simulink model "buck_converter_with_Hysteresis_control"  (R2015a)
settings: Solver=ode45  StartTime=0.0  StopTime=3/1000  MaxStep=1/1000000  RelTol=1e-3
libraries: powerlib x9
settings Model: Creator=Windows 10  LastModifiedBy=Windows 10

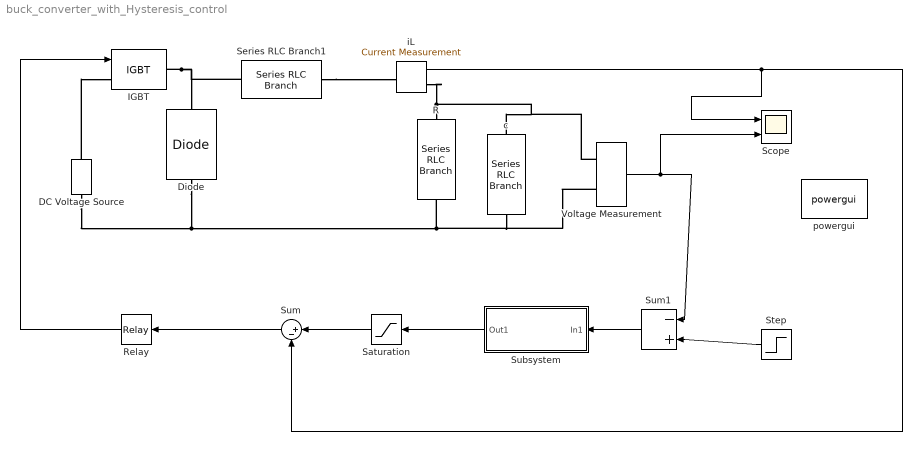
== system buck_converter_with_Hysteresis_control ==
  DC Voltage Source : powerlib/Electrical Sources/DC Voltage Source  Amplitude=100  Measurements=None
  Diode : powerlib/Power Electronics/Diode  Ron=0.001  Lon=0  Vf=0.8  IC=0  UseSnubber=off  Rs=500  Cs=250e-9  Measurements=off
  IGBT : powerlib/Power Electronics/IGBT  Ron=0.001  Lon=0  Vf=1  Tf=1e-6  Tt=2e-6  IC=0  Rs=1e5  Cs=inf  Measurements=off
  R : powerlib/Elements/Series RLC Branch  LConnTagsString=__new0  RConnTagsString=__new0  BranchType=R  Resistance=5  Inductance=1e-3  SetiL0=off  InitialCurrent=0  Capacitance=1e-6  Setx0=off  InitialVoltage=0  Measurements=None
  Relay : Relay  OnSwitchValue=0.5  OffSwitchValue=-0.5
  Saturation : Saturate  UpperLimit=20  LowerLimit=-20
  Scope : Scope  NumInputPorts=2
      settings: YMin=-5~-5  YMax=5~5
  Series RLC Branch1 : powerlib/Elements/Series RLC Branch  LConnTagsString=__new0  RConnTagsString=__new0  BranchType=L  Resistance=5  Inductance=0.01e-3  SetiL0=off  InitialCurrent=0  Capacitance=1e-6  Setx0=off  InitialVoltage=0  Measurements=Branch voltage
  Step : Step  Time=1.5/1000  Before=50  After=80  SampleTime=0
  Subsystem : Subsystem
  Sum : Sum  Inputs=|+-
  Sum1 : Sum  Inputs=|-+
  Voltage Measurement : powerlib/Measurements/Voltage Measurement  PhasorSimulation=off  OutputType=Complex  PSBequivalent=0
  c : powerlib/Elements/Series RLC Branch  LConnTagsString=__new0  RConnTagsString=__new0  BranchType=C  Resistance=5  Inductance=1e-3  SetiL0=off  InitialCurrent=0  Capacitance=20e-6  Setx0=off  InitialVoltage=0  Measurements=None
  iL : powerlib/Measurements/Current Measurement  PhasorSimulation=off  OutputType=Complex  PSBequivalent=0
  powergui : powerlib/powergui  Priority=1  SimulationMode=Continuous  SolverType=Tustin/Backward Euler (TBE)  SampleTime=50e-6  frequency=60  SPID=off  DisableSnubberDevices=off  DisableRonSwitches=off  DisableVfSwitches=off  SwTol=0  DisplayEquations=off  Interpol=off  methode=off  Ts=100  FunctionMessages=off  echomessages=off  HookPort=off  EnableUseOfTLC=off  x0status=blocks  frequencyindice=0  Pbase=100e6  ErrMax=1e-4  Iterations=50  UnitsV=kV  UnitsW=MW  buscounter=0  RestoreLinks=warning  ResistiveCurrentMeasurement=off  Frange=[0:2:500]  Ylog=off  Xlog=on  ShowGrid=off  save=off  variable=ZData  structure=0  ZoomFFT=off  StartTime=0.0  cycles=1  DisplayStyle=1  fundamental=60  FreqAxis=off  MaxFrequency=1000  frequencyindicesteady=1  RmsSteady=1  display=off
  wires:
  iL/1 -> Sum/2, Scope/1
  Voltage Measurement/1 -> Sum1/1, Scope/2
  Relay/1 -> IGBT/1
  Step/1 -> Sum1/2
  Sum/1 -> Relay/1
  Sum1/1 -> Subsystem/1(In1)
  Subsystem/1(Out1) -> Saturation/1
  Saturation/1 -> Sum/1
  connections:
  DC Voltage Source/RConn1 -- IGBT/LConn1
  IGBT/RConn1 -- Series RLC Branch1/RConn1 -- Diode/RConn1
  DC Voltage Source/LConn1 -- Voltage Measurement/LConn2 -- c/RConn1 -- R/RConn1 -- Diode/LConn1
  iL/RConn1 -- c/LConn1 -- Voltage Measurement/LConn1 -- R/LConn1
  Series RLC Branch1/LConn1 -- iL/LConn1

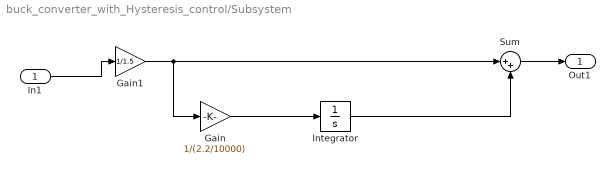
== system buck_converter_with_Hysteresis_control/Subsystem ==
  In1 : Inport
  Gain : Gain  Gain=1/(2.2/10000)
  Gain1 : Gain  Gain=1/1.5
  Integrator : Integrator
  Sum : Sum  Inputs=|++
  Out1 : Outport
  wires:
  In1/1 -> Gain1/1
  Gain/1 -> Integrator/1
  Integrator/1 -> Sum/2
  Gain1/1 -> Sum/1, Gain/1
  Sum/1 -> Out1/1
